simulink model "waypoints_pid"  (R2024a)
settings: Solver=VariableStepAuto  StartTime=0.0  StopTime=inf  RelTol=1e-3
undefined symbols (not defined in the file or in its folder): Angular, Linear
libraries: robotlib x3, slpidlib x1
settings Model: Creator=auvsl  LastModifiedBy=auvsl

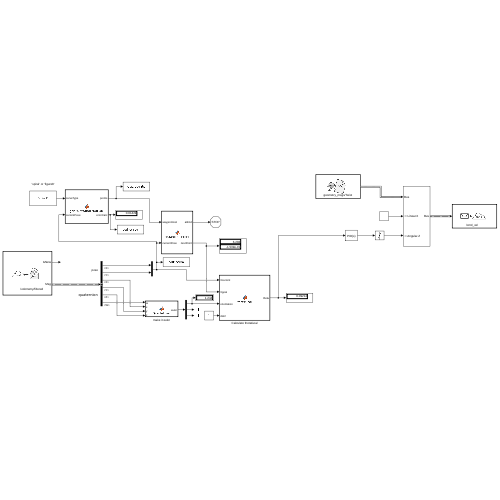
[thumbnail: Simulink's stored preview of the top-level diagram]
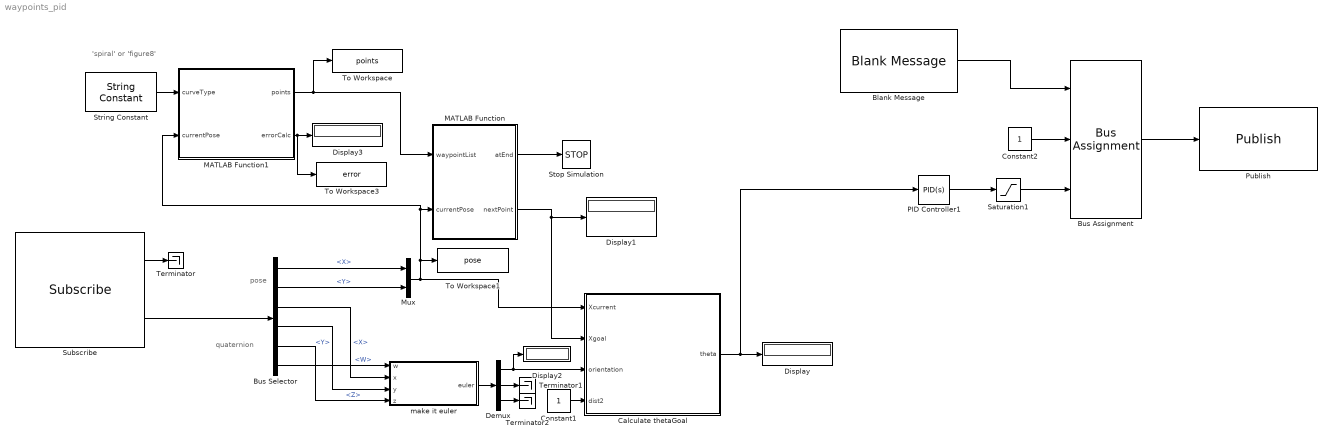
== system waypoints_pid ==
  note: 'spiral' or 'figure8'
  note: pose
  note: quaternion
  Blank Message : robotlib/Blank Message  messageClass=Message  entityType=geometry_msgs/Twist  messageType=geometry_msgs/Twist  SampleTime=inf  legacyBusStruct=off
  Bus Assignment : BusAssignment  AssignedSignals=Linear.X,Angular.Z
  Bus Selector : BusSelector  OutputSignals=Pose.Pose.Position.X,Pose.Pose.Position.Y,Pose.Pose.Orientation.X,Pose.Pose.Orientation.Y,Pose.Pose.Orientation.Z,Pose.Pose.Orientation.W
  Calculate thetaGoal : MATLAB Function  TreatAsAtomicUnit=on
  Constant1 : Constant
  Constant2 : Constant
  Demux : Demux  Outputs=3
  Display{,1..3} (4 alike) : Display
  MATLAB Function : MATLAB Function  TreatAsAtomicUnit=on
  MATLAB Function1 : MATLAB Function  TreatAsAtomicUnit=on
  Mux : Mux  Inputs=2
  PID Controller1 : slpidlib/PID Controller  Controller=PID  Form=Parallel  TimeDomain=Continuous-time  UseExternalTs=off  SampleTime=-1  IntegratorMethod=Forward Euler  FilterMethod=Forward Euler  ControllerParametersSource=internal  P=20e-1  I=0  UseKiTs=off  D=0.3  UseExternalDerivativeSource=off  N=100  UseFilter=on  TunerSelectOption=Transfer Function Based (PID Tuner App)  InitialConditionSource=internal  InitialConditionForIntegrator=0  InitialConditionForFilter=0  DifferentiatorICPrevScaledInput=0  ExternalReset=none  TrackingMode=off  Kt=1  LimitOutput=off  SatLimitsSource=internal  UpperSaturationLimit=inf  LowerSaturationLimit=-inf  LinearizeAsGain=on  AntiWindupMode=none  Kb=1  LimitIntegrator=off  UpperIntegratorSaturationLimit=inf  LowerIntegratorSaturationLimit=-inf  POutMin=[]  POutMax=[]  IOutMin=[]  IOutMax=[]  DOutMin=[]  DOutMax=[]  NOutMin=[]  NOutMax=[]  SumOutMin=[]  SumOutMax=[]  SaturationOutMin=[]  SaturationOutMax=[]  PParamMin=[]  PParamMax=[]  IParamMin=[]  IParamMax=[]  DParamMin=[]  DParamMax=[]  NParamMin=[]  NParamMax=[]  KbParamMin=[]  KbParamMax=[]  KtParamMin=[]  KtParamMax=[]  KbOutMin=[]  KbOutMax=[]  KtOutMin=[]  KtOutMax=[]  IntegratorOutMin=[]  IntegratorOutMax=[]  FilterOutMin=[]  FilterOutMax=[]  SumI1OutMin=[]  SumI1OutMax=[]  SumI2OutMin=[]  SumI2OutMax=[]  SumI3OutMin=[]  SumI3OutMax=[]  SumI4OutMin=[]  SumI4OutMax=[]  SumDOutMin=[]  SumDOutMax=[]  DifferentiatorOutMin=[]  DifferentiatorOutMax=[]  FilterDiffOutCoefMin=[]  FilterDiffOutCoefMax=[]  ReciprocalOutMin=[]  ReciprocalOutMax=[]  SumDenOutMin=[]  SumDenOutMax=[]  SumNumOutMin=[]  SumNumOutMax=[]  DivideOutMin=[]  DivideOutMax=[]  UdiffTsProdOutMin=[]  UdiffTsProdOutMax=[]  NTsProdOutMin=[]  NTsProdOutMax=[]  UintegralTsProdOutMin=[]  UintegralTsProdOutMax=[]  UngainTsProdOutMin=[]  UngainTsProdOutMax=[]  ClampingZeroOutDataTypeStr=Inherit: Inherit via back propagation  ClampingZeroOutMin=[]  ClampingZeroOutMax=[]  FilterDenConstantOutDataTypeStr=Inherit: Inherit via back propagation  FilterDenConstantOutMin=[]  FilterDenConstantOutMax=[]  PCopyOutDataTypeStr=Inherit: Inherit via back propagation  PCopyOutMin=[]  PCopyOutMax=[]  NCopyOutDataTypeStr=Inherit: Inherit via back propagation  NCopyOutMin=[]  NCopyOutMax=[]  IntegratorContinuousStateAttributes=''  IntegratorStateMustResolveToSignalObject=off  IntegratorRTWStateStorageClass=Auto  FilterContinuousStateAttributes=''  FilterStateMustResolveToSignalObject=off  FilterRTWStateStorageClass=Auto  ParallelPVariant=InternalParameters  IdealPVariant=Disabled  IVariant=InternalParameters  DVariant=InternalParameters  IntegratorVariant=Continuous  SatVariant=Disabled  AWVariant=Passthrough  PCopyVariant=Disabled  TRVariant=Disabled  FdbkBlocksVariant=Forward  IdealPFdbkVariant=Disabled  SatFdbkVariant=Disabled  DerivativeFilterVariant=ContFilter  NVariant=InternalParameters  NCopyVariant=Disabled  FilterICVariant=InternalICsFilter  IntegratorICVariant=InternalICs  ExternalResetVariant=Disabled  TRSumVariant=Passthrough  SumFdbkVariant=Disabled  SumVariant=Sum_PID  TsampFilterVariant=InternalTs  TsampNgainVariant=Passthrough  TsampIntegralVariant=Disabled_SignalSpec  ExternalSaturationOutDataTypeStr=Inherit: Same as second input  DerivativeSourceVariant=ErrorSignal
  Publish : robotlib/Publish  topicSource=Select from ROS network  topic=/cmd_vel  messageType=geometry_msgs/Twist  legacyBusStruct=off  messageQueueLength=1
  Saturation1 : Saturate  UpperLimit=2  LowerLimit=-2
  Stop Simulation : Stop
  String Constant : StringConstant  String='spiral'
  Subscribe : robotlib/Subscribe  topicSource=Select from ROS network  topic=/odometry/filtered  messageType=nav_msgs/Odometry  SampleTime=-1  legacyBusStruct=off  messageQueueLength=1
  Terminator : Terminator
  Terminator1 : Terminator
  Terminator2 : Terminator
  To Workspace : ToWorkspace  VariableName=points  SaveFormat=Timeseries  SampleTime=-1
  To Workspace1 : ToWorkspace  VariableName=pose  SaveFormat=Timeseries  SampleTime=-1
  To Workspace3 : ToWorkspace  VariableName=error  SaveFormat=Timeseries  SampleTime=-1
  make it euler : MATLAB Function  TreatAsAtomicUnit=on
  wires:
  Bus Selector/6 -> make it euler/1(w)  "<W>"
  Bus Selector/2 -> Mux/2  "<Y>"
  make it euler/1(euler) -> Demux/1
  Mux/1 -> MATLAB Function1/2(currentPose), MATLAB Function/2(currentPose), To Workspace1/1, Calculate thetaGoal/1(Xcurrent)
  Bus Selector/4 -> make it euler/3(y)  "<Y>"
  Calculate thetaGoal/1(theta) -> PID Controller1/1, Display/1
  Constant1/1 -> Calculate thetaGoal/4(dist2)
  Demux/2 -> Terminator1/1
  Bus Selector/5 -> make it euler/4(z)  "<Z>"
  Demux/1 -> Display2/1, Calculate thetaGoal/3(orientation)
  MATLAB Function/2(nextPoint) -> Calculate thetaGoal/2(Xgoal), Display1/1
  Bus Selector/3 -> make it euler/2(x)  "<X>"
  Demux/3 -> Terminator2/1
  Subscribe/2 -> Bus Selector/1
  Bus Selector/1 -> Mux/1  "<X>"
  Subscribe/1 -> Terminator/1
  Bus Assignment/1 -> Publish/1
  Blank Message/1 -> Bus Assignment/1
  Constant2/1 -> Bus Assignment/2
  Saturation1/1 -> Bus Assignment/3
  PID Controller1/1 -> Saturation1/1
  MATLAB Function1/1(points) -> To Workspace/1, MATLAB Function/1(waypointList)
  MATLAB Function1/2(errorCalc) -> To Workspace3/1, Display3/1
  String Constant/1 -> MATLAB Function1/1(curveType)
  MATLAB Function/1(atEnd) -> Stop Simulation/1

== matlab function waypoints_pid/Calculate thetaGoal ==
  data: Xcurrent input; theta output; Xgoal input; orientation input; dist2 input
function theta = thetaGoal(Xcurrent, Xgoal, orientation, dist2)

Xcurrent = transpose(Xcurrent);
Xtrans = Xgoal-Xcurrent;
thetatrans = atan2(Xtrans(2), Xtrans(1));

theta = thetatrans - orientation;

% added to stop weird behavior due to theta changing quickly close to goal
if dist2 < 0.1
    theta = 0;
end

% trying to restrict to -pi < theta < pi
if theta > pi
    theta = theta - 2*pi;
elseif theta < -pi
    theta = theta + 2*pi;
end

== matlab function waypoints_pid/make it euler ==
  data: w input; euler output; x input; y input; z input
function euler = QuatToEuler(w, x, y, z)
%#codegen

quat = [w x y z];

if quat == [0 0 0 0]
    quat = [1 0 0 0];
end

euler = quat2eul(quat);

== matlab function waypoints_pid/MATLAB Function ==
  data: atEnd output; waypointList input; nextPoint output; currentPose input
function [atEnd, nextPoint] = distanceChecker(waypointList, currentPose)

persistent count

if isempty(count)
    count = 1;
end

nextPoint = waypointList(count, :);

atEnd = 0;
if count == length(waypointList) % & dotproduct < threshold
    atEnd = 1
end

currentGoal = waypointList(count, :);
currentPose = transpose(currentPose);

diff = currentPose - currentGoal;
dotproduct = dot(diff, diff);
threshold = 0.1;

if dotproduct < threshold
    count = count + 1;
end



end

== matlab function waypoints_pid/MATLAB Function1 ==
  data: curveType input; points output; errorCalc output; currentPose input
function [points, errorCalc] = genPointsAndErrorCalc(curveType, currentPose)
num_points = 50;

t = linspace(0, 2*pi, num_points);
x = 5 * sin(t);
y = 5 * sin(t) .* cos(t); % defined x and y here otherwise it gives me an error


spiralSize = 2*pi;

if strcmp(curveType, 'figure8')
    t = linspace(0, 2*pi, num_points);
    x = 5 * sin(t);
    y = 5 * sin(t) .* cos(t);
elseif strcmp(curveType, 'spiral')
    t = linspace(0, spiralSize, num_points);
    x = t .* cos(t);
    y = t .* sin(t);
else
    error('unknown curve type')
end

points = [x' y'];

% yeah
currentPose = transpose(currentPose)

% make some variables before giving them values in the if statement
t_min = 1;
fval = 0;

% emmpty variables for spiral error
checkSize = pi/6;
checkNum = floor(spiralSize / checkSize)
bounds = zeros(1, checkNum+1); % bc 13 endpoints means 12 intervals
vals = zeros(1, checkNum);
v_min = 2;

% find time when the closest point occurs
if strcmp(curveType, 'figure8')
    distance_square = @(t) (currentPose(1) - 5 * sin(t)).^2 + (currentPose(2) - 5 * sin(t) .* cos(t)).^2 ; 
    [t_min, fval] = fminbnd(distance_square, 0, 2*pi);
    v_min = fval;
elseif strcmp(curveType, 'spiral')
    distance_square = @(t) (currentPose(1) - t .* cos(t)).^2 + (currentPose(2) - t .* sin(t)).^2 ;
    for i = 1:checkNum+1
        bounds(i) = checkSize*(i-1);
    end

    for i = 1:checkNum
        [t_min_candidate, fval] = fminbnd(distance_square, bounds(i) , bounds(i+1));
        vals(i) = fval;
    end

    v_min = min(vals);    

end

errorCalc = sqrt(v_min);

end
